simulink model "Simula_Maq_1"  (R2017a)
settings: Solver=VariableStepAuto  StartTime=0.0  StopTime=1/30  MaxStep=1e-4  RelTol=1e-3
values from neighbouring files (symbols this model uses):
  R = 0    [Simul_trans1.m]
libraries: fl_lib x17, nesl_utility x7
settings Model: Creator=gabriel  LastModifiedBy=gabriel

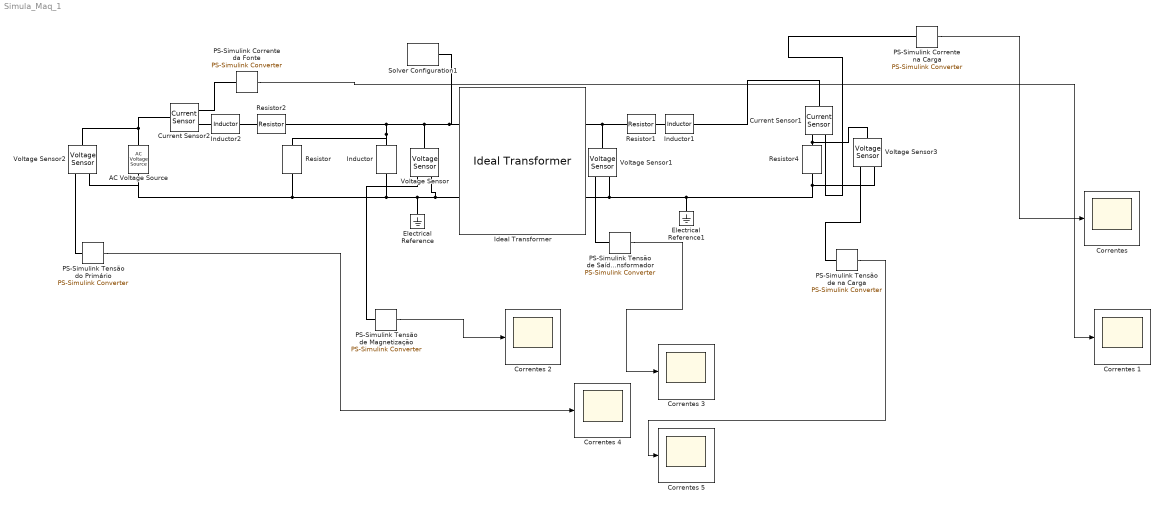
== system Simula_Maq_1 ==
  AC Voltage Source : fl_lib/Electrical/Electrical Sources/AC Voltage Source  amp=220*1.4 V  shift=0 deg  frequency=60 Hz  omega=0 rad/s
  Correntes {,1..5} (6 alike) : Scope
  Current Sensor1 : fl_lib/Electrical/Electrical Sensors/Current Sensor
  Current Sensor2 : fl_lib/Electrical/Electrical Sensors/Current Sensor
  Electrical Reference : fl_lib/Electrical/Electrical Elements/Electrical Reference
  Electrical Reference1 : fl_lib/Electrical/Electrical Elements/Electrical Reference
  Ideal Transformer : fl_lib/Electrical/Electrical Elements/Ideal Transformer  n=2  i1_specify=off  i1_priority=None  i1=0 A  i1_nominal_specify=off  i1_nominal_unit=A  i1_nominal_value=1  v1_specify=off  v1_priority=None  v1=0 V  v1_nominal_specify=off  v1_nominal_unit=V  v1_nominal_value=1  i2_specify=off  i2_priority=None  i2=0 A  i2_nominal_specify=off  i2_nominal_unit=A  i2_nominal_value=1  v2_specify=off  v2_priority=None  v2=0 V  v2_nominal_specify=off  v2_nominal_unit=V  v2_nominal_value=1
      settings: SourceProductName=Simscape  SourceProductBaseCode=SS
  Inductor : fl_lib/Electrical/Electrical Elements/Inductor  l=2000/(2*pi*60) H  r=0 Ohm  g=1e-9 1/Ohm  i_specify=off  i_priority=None  i=0 A  i_nominal_specify=off  i_nominal_unit=A  i_nominal_value=1  v_specify=off  v_priority=None  v=0 V  v_nominal_specify=off  v_nominal_unit=V  v_nominal_value=1  i_L_specify=off  i_L_priority=High  i_L=0 A  i_L_nominal_specify=off  i_L_nominal_unit=A  i_L_nominal_value=1
  Inductor1 : fl_lib/Electrical/Electrical Elements/Inductor  l=100/(2*pi*60) H  r=0 Ohm  g=1e-9 1/Ohm  i_specify=off  i_priority=None  i=0 A  i_nominal_specify=off  i_nominal_unit=A  i_nominal_value=1  v_specify=off  v_priority=None  v=0 V  v_nominal_specify=off  v_nominal_unit=V  v_nominal_value=1  i_L_specify=off  i_L_priority=High  i_L=0 A  i_L_nominal_specify=off  i_L_nominal_unit=A  i_L_nominal_value=1
  Inductor2 : fl_lib/Electrical/Electrical Elements/Inductor  l=100/(2*pi*60) H  r=0 Ohm  g=1e-9 1/Ohm  i_specify=off  i_priority=None  i=0 A  i_nominal_specify=off  i_nominal_unit=A  i_nominal_value=1  v_specify=off  v_priority=None  v=0 V  v_nominal_specify=off  v_nominal_unit=V  v_nominal_value=1  i_L_specify=off  i_L_priority=High  i_L=0 A  i_L_nominal_specify=off  i_L_nominal_unit=A  i_L_nominal_value=1
  PS-Simulink Corrente da Fonte : nesl_utility/PS-Simulink Converter  PhysicalDomain=network_engine_domain  SubClassName=ps_output  LeftPortType=input  RightPortType=output  PseudoPeriodic=off  Frequencies=[]  Unit=1  AffineConversion=off
  "PS-Simulink Corrente na Carga " : nesl_utility/PS-Simulink Converter  PhysicalDomain=network_engine_domain  SubClassName=ps_output  LeftPortType=input  RightPortType=output  PseudoPeriodic=off  Frequencies=[]  Unit=1  AffineConversion=off
  "PS-Simulink Tensão de Magnetização " : nesl_utility/PS-Simulink Converter  PhysicalDomain=network_engine_domain  SubClassName=ps_output  LeftPortType=input  RightPortType=output  PseudoPeriodic=off  Frequencies=[]  Unit=1  AffineConversion=off
  "PS-Simulink Tensão de Saída do Transformador " : nesl_utility/PS-Simulink Converter  PhysicalDomain=network_engine_domain  SubClassName=ps_output  LeftPortType=input  RightPortType=output  PseudoPeriodic=off  Frequencies=[]  Unit=1  AffineConversion=off
  "PS-Simulink Tensão de na Carga " : nesl_utility/PS-Simulink Converter  PhysicalDomain=network_engine_domain  SubClassName=ps_output  LeftPortType=input  RightPortType=output  PseudoPeriodic=off  Frequencies=[]  Unit=1  AffineConversion=off
  "PS-Simulink Tensão do Primário " : nesl_utility/PS-Simulink Converter  PhysicalDomain=network_engine_domain  SubClassName=ps_output  LeftPortType=input  RightPortType=output  PseudoPeriodic=off  Frequencies=[]  Unit=1  AffineConversion=off
  Resistor : fl_lib/Electrical/Electrical Elements/Resistor  R=1000 Ohm  i_specify=off  i_priority=None  i=0 A  i_nominal_specify=off  i_nominal_unit=A  i_nominal_value=1  v_specify=off  v_priority=None  v=0 V  v_nominal_specify=off  v_nominal_unit=V  v_nominal_value=1
  Resistor1 : fl_lib/Electrical/Electrical Elements/Resistor  R=10 Ohm  i_specify=off  i_priority=None  i=0 A  i_nominal_specify=off  i_nominal_unit=A  i_nominal_value=1  v_specify=off  v_priority=None  v=0 V  v_nominal_specify=off  v_nominal_unit=V  v_nominal_value=1
  Resistor2 : fl_lib/Electrical/Electrical Elements/Resistor  R=10 Ohm  i_specify=off  i_priority=None  i=0 A  i_nominal_specify=off  i_nominal_unit=A  i_nominal_value=1  v_specify=off  v_priority=None  v=0 V  v_nominal_specify=off  v_nominal_unit=V  v_nominal_value=1
  Resistor4 : fl_lib/Electrical/Electrical Elements/Resistor  R=R Ohm  i_specify=off  i_priority=None  i=0 A  i_nominal_specify=off  i_nominal_unit=A  i_nominal_value=1  v_specify=off  v_priority=None  v=0 V  v_nominal_specify=off  v_nominal_unit=V  v_nominal_value=1
  Solver Configuration1 : nesl_utility/Solver Configuration  PhysicalDomain=network_engine_domain  SubClassName=solver  LeftPortType=input  RightPortType=generic  Accelerate=off  Tones=[]  Harmonics=[]  SimulateNoise=off  Profile=off  UseLocalSampling=off  EnableSwitchedLinearOptims=on  FrequencyDomain=off  UseCCode=off  RelTol=0.001  AbsTol=1e-06  MinStep=1e-09  ToWorkspace=off  RevertToSquareIcSolve=off  NumHomotopyIterations=100  PhasorMode=off  PhasorModeNumHarmonics=1  OverrideAbsTol=off  DoDC=off  ResidualTolerance=1e-09  UseLocalSolver=off  LocalSolverChoice=NE_BACKWARD_EULER_ADVANCER  LocalSolverSampleTime=0.001  DoFixedCost=off  MaxNonlinIter=3  MaxModeIter=2  LinearAlgebra=Sparse  DelaysMemoryBudget=1024  AutomaticFiltering=on  FilteringTimeConstant=0.001
  Voltage Sensor{,1..3} (4 alike) : fl_lib/Electrical/Electrical Sensors/Voltage Sensor
  wires:
  "PS-Simulink Tensão de Magnetização "/1 -> Correntes 2/1
  "PS-Simulink Tensão do Primário "/1 -> Correntes 4/1
  "PS-Simulink Tensão de na Carga "/1 -> Correntes 5/1
  "PS-Simulink Corrente na Carga "/1 -> "Correntes "/1
  PS-Simulink Corrente da Fonte/1 -> Correntes 1/1
  "PS-Simulink Tensão de Saída do Transformador "/1 -> Correntes 3/1
  connections:
  Inductor/LConn1 -- Resistor/LConn1 -- Voltage Sensor/LConn1 -- Solver Configuration1/RConn1 -- Ideal Transformer/LConn1 -- Resistor2/RConn1
  Inductor/RConn1 -- Voltage Sensor2/RConn2 -- AC Voltage Source/RConn1 -- Resistor/RConn1 -- Electrical Reference/LConn1 -- Voltage Sensor/RConn2 -- Ideal Transformer/LConn2
  Resistor1/LConn1 -- Voltage Sensor1/LConn1 -- Ideal Transformer/RConn1
  Inductor1/LConn1 -- Resistor1/RConn1
  Resistor4/RConn1 -- Voltage Sensor3/RConn2 -- Electrical Reference1/LConn1 -- Voltage Sensor1/RConn2 -- Ideal Transformer/RConn2
  Inductor2/RConn1 -- Resistor2/LConn1
  Voltage Sensor2/LConn1 -- AC Voltage Source/LConn1 -- Current Sensor2/LConn1
  Voltage Sensor/RConn1 -- "PS-Simulink Tensão de Magnetização "/LConn1
  Voltage Sensor1/RConn1 -- "PS-Simulink Tensão de Saída do Transformador "/LConn1
  Voltage Sensor2/RConn1 -- "PS-Simulink Tensão do Primário "/LConn1
  Current Sensor2/RConn2 -- Inductor2/LConn1
  Current Sensor2/RConn1 -- PS-Simulink Corrente da Fonte/LConn1
  Current Sensor1/LConn1 -- Inductor1/RConn1
  Current Sensor1/RConn2 -- Voltage Sensor3/LConn1 -- Resistor4/LConn1
  Current Sensor1/RConn1 -- "PS-Simulink Corrente na Carga "/LConn1
  Voltage Sensor3/RConn1 -- "PS-Simulink Tensão de na Carga "/LConn1
